simulink model "gm_hdlcoder_led_blinking_4bit_interface"  (R2021b)
settings: Solver=FixedStepDiscrete  StartTime=0.0  StopTime=inf  RelTol=1e-3  EnableMultiTasking=on
InitFcn:
  | Ts = 1e-3;
undefined symbols (not defined in the file or in its folder): AXI4, Lite
libraries: axiinterfacelib x3, simulink x2
settings Model: Creator=The MathWorks, Inc.  LastModifiedBy=Jeedella
settings SolverCC: ConcurrentTasks=on  AlgebraicLoopSolver=TrustRegion  PositivePriorityOrder=on
settings DataIOCC: LimitDataPoints=on  SaveFormat=Array  SaveOutput=off  SignalLogging=off  SaveTime=off  ReturnWorkspaceOutputs=off
settings OptimizationCC: BlockReduction=off  ConditionallyExecuteInputs=off  EnhancedBackFolding=on  PassReuseOutputArgsAs=Individual arguments  ExpressionDepthLimit=2147483647  ZeroExternalMemoryAtStartup=off  ZeroInternalMemoryAtStartup=off  MaxStackSize=64  OptimizeBlockOrder=speed  DifferentSizesBufferReuse=on  OptimizationCustomize=off  EfficientTunableParamExpr=on
settings DebuggingCC: AlgebraicLoopMsg=error  UnderspecifiedInitializationDetection=Classic  MergeDetectMultiDrivingBlocksExec=none  SolverPrmCheckMsg=warning  SingleTaskRateTransMsg=error  ParameterPrecisionLossMsg=none  ParameterTunabilityLossMsg=error  StateNameClashWarn=warning  SFUnexpectedBacktrackingDiag=warning  SFNoUnconditionalDefaultTransitionDiag=warning  SFExecutionAtInitializationDiag=none  SFMachineParentedDataDiag=warning  ArithmeticOperatorsInVariantConditions=warning
settings HardwareCC: ProdBitPerPointer=32  ProdBitPerSizeT=32  ProdBitPerPtrDiffT=32  ProdLargestAtomicInteger=Long  ProdLargestAtomicFloat=Double  ProdWordSize=32  ProdLongLongMode=on  ProdHWDeviceType=ARM Compatible->ARM Cortex  TargetEndianess=LittleEndian
settings ModelReferenceCC: ModelReferenceNumInstancesAllowed=Single  PropagateSignalLabelsOutOfModel=off
settings SFSimCC: SimUseLocalCustomCode=off  MATLABDynamicMemAlloc=off  CustomCodeUndefinedFunction=UseInterfaceOnly
settings RTWCC: Description=Embedded Coder  SystemTargetFile=ert.tlc  HardwareBoard=Xilinx Zynq-7000 based board  TLCOptions="-aInlineSetEventsForThisBaseRateFcn=TLC_FALSE -aSuppressMultiTaskScheduler=TLC_FALSE  -aRateBasedStepFcn=0"  TemplateMakefile=ert_default_tmf  RTWUseLocalCustomCode=off  Toolchain=Linaro AArch32 Linux v6.3.1
settings CodeAppCC: ForceParamTrailComments=on  IgnoreCustomStorageClasses=off  OperatorAnnotations=on  SimulinkDataObjDesc=on  SFDataObjDesc=on  InsertBlockDesc=on
settings ConfigComp: CovMetricSettings=dw  CovSaveCumulativeToWorkspaceVar=on  CovSaveSingleToWorkspaceVar=on  CovExternalEMLEnable=off  CovSFcnEnable=off

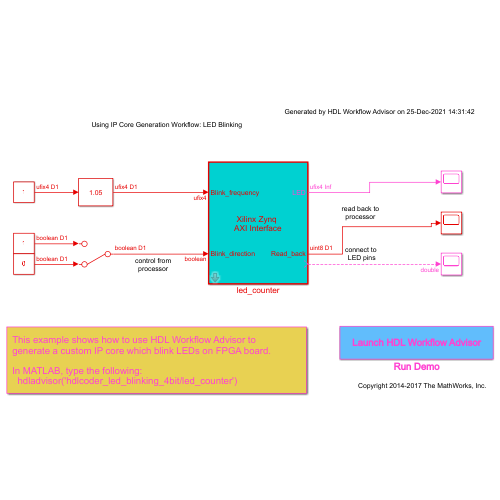
[thumbnail: Simulink's stored preview of the top-level diagram]
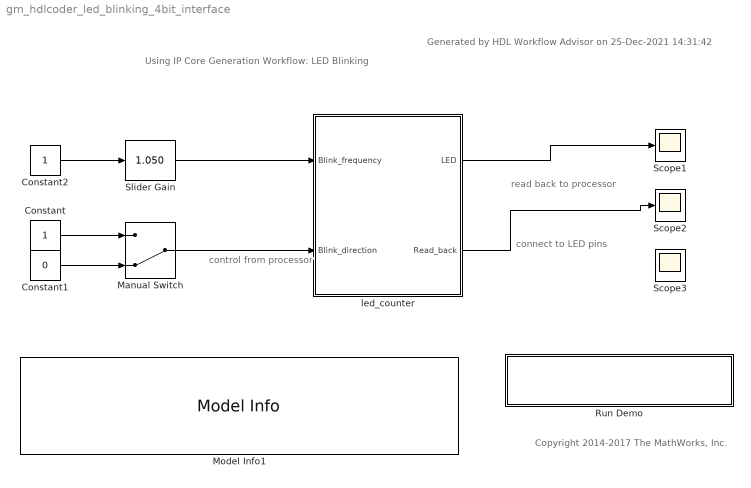
== system gm_hdlcoder_led_blinking_4bit_interface ==
  note: connect to
      | LED pins
  note: read back to
      | processor
  note: control from
      | processor
  note: Using IP Core Generation Workflow: LED Blinking
  note: Copyright 2014-2017 The MathWorks, Inc.
  note: Generated by HDL Workflow Advisor on 25-Dec-2021 14:31:42
  Constant : Constant  OutDataTypeStr=boolean  SampleTime=Ts
  Constant1 : Constant  Value=0  OutDataTypeStr=boolean  SampleTime=Ts
  Constant2 : Constant  OutDataTypeStr=fixdt(0, 4, 0)  SampleTime=Ts
  Manual Switch : ManualSwitch  CurrentSetting=0
  Model Info1 : simulink/Model-Wide Utilities/Model Info  Frame=on  DisplayStringWithTags=|  HorizontalTextAlignment=Left  LeftAlignmentValue=0.02
      | This example shows how to use HDL Workflow Advisor to    
      | generate a custom IP core which blink LEDs on FPGA board.
      |                                                          
      | In MATLAB, type the following:                           
      |   hdladvisor('hdlcoder_led_blinking_4bit/led_counter')
  Run Demo : Subsystem
      settings: OpenFcn=hdladvisor([bdroot, '/led_counter'])
      mask Display: disp('Launch HDL Workflow Advisor')
  Scope1 : Scope
  Scope2 : Scope
  Scope3 : Scope
  Slider Gain : simulink/Math Operations/Slider Gain  gain=1.050  low=0  high=15
  led_counter : Subsystem  TreatAsAtomicUnit=on  mask(AXI4-Lite/AXI4 Interface){}
      mask help:
      | This is an automatically generated subsystem block.
      | This contains the AXI interface blocks that communicate with the led_count_ip IPCore generated from hdlcoder_led_blinking_4bit/led_counter subsystem.
      mask Display: disp(sprintf('Xilinx Zynq \nAXI Interface'));
  wires:
  ? -> Scope3/1
  led_counter/1(LED) -> Scope1/1
  led_counter/2(Read_back) -> Scope2/1
  Slider Gain/1 -> led_counter/1(Blink_frequency)
  Constant2/1 -> Slider Gain/1
  Manual Switch/1 -> led_counter/2(Blink_direction)
  Constant1/1 -> Manual Switch/2
  Constant/1 -> Manual Switch/1

== system gm_hdlcoder_led_blinking_4bit_interface/Run Demo ==

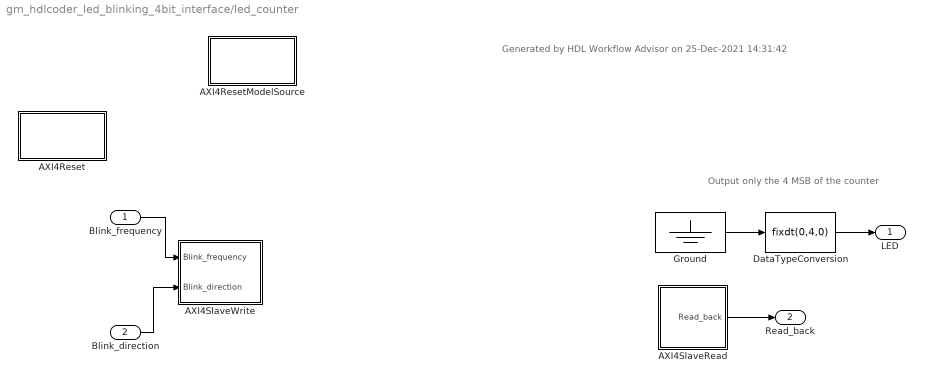
== system gm_hdlcoder_led_blinking_4bit_interface/led_counter ==
  note: Output only the 4 MSB of the counter
  note: Generated by HDL Workflow Advisor on 25-Dec-2021 14:31:42
  Blink_frequency : Inport  OutDataTypeStr=fixdt(0, 4, 0)
  Blink_direction : Inport  Port=2  OutDataTypeStr=boolean
  AXI4Reset : Subsystem  mask(System Start){ShowInLibBrowser=0}
      mask prompts: ShowInLibBrowser "Simulink:masks:CustCodeMaskParam1_MP"
      settings: CopyFcn=cccopyfcn(gcb)  OpenFcn=ccopenfcn('System Start Function')
      mask Help: eval('feval(''rtwprivate'',''rtwhelpview'',''rtw_sys_start_block'')');
      mask Display: disp('System\nStart');
  AXI4ResetModelSource : Subsystem  mask(Model Source){ShowInLibBrowser=0}
      mask prompts: ShowInLibBrowser "Simulink:masks:CustCodeMaskParam1_MP"
      settings: CopyFcn=cccopyfcn(gcb)  OpenFcn=ccopenfcn('Model Source')
      mask Help: eval('feval(''rtwprivate'',''rtwhelpview'',''rtw_model_source_block'')');
      mask Display: disp('Model\nSource');
  AXI4SlaveRead : Subsystem  Priority=10
  AXI4SlaveWrite : Subsystem  Priority=1
  DataTypeConversion : DataTypeConversion  OutDataTypeStr=fixdt(0,4,0)  ConvertRealWorld=Stored Integer (SI)
  Ground : Ground
  LED : Outport  VectorParamsAs1DForOutWhenUnconnected=off
  Read_back : Outport  Port=2  VectorParamsAs1DForOutWhenUnconnected=off
  wires:
  Blink_frequency/1 -> AXI4SlaveWrite/1(Blink_frequency)
  Blink_direction/1 -> AXI4SlaveWrite/2(Blink_direction)
  AXI4SlaveRead/1(Read_back) -> Read_back/1
  DataTypeConversion/1 -> LED/1
  Ground/1 -> DataTypeConversion/1

== system gm_hdlcoder_led_blinking_4bit_interface/led_counter/AXI4Reset ==

== system gm_hdlcoder_led_blinking_4bit_interface/led_counter/AXI4ResetModelSource ==

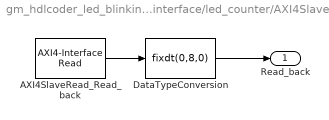
== system gm_hdlcoder_led_blinking_4bit_interface/led_counter/AXI4SlaveRead ==
  AXI4SlaveRead_Read_back : axiinterfacelib/AXI4-Interface Read  Priority=3  AXIInterfaceType=AXI4-Lite  DeviceName=/dev/mwipcore  RegisterOffset=hex2dec('108')  DataLength=1  DataType=uint32  SampleTime=-1  blockPlatform=ZYNQ  SimulateUsing=Interpreted Execution
      settings: SourceProductBaseCode=ECZYNQ7000
  DataTypeConversion : DataTypeConversion  OutDataTypeStr=fixdt(0,8,0)  ConvertRealWorld=Stored Integer (SI)
  Read_back : Outport  VectorParamsAs1DForOutWhenUnconnected=off
  wires:
  DataTypeConversion/1 -> Read_back/1
  AXI4SlaveRead_Read_back/1 -> DataTypeConversion/1

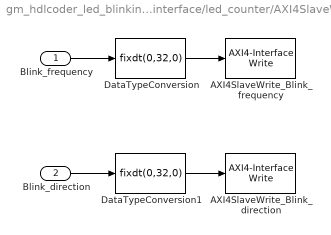
== system gm_hdlcoder_led_blinking_4bit_interface/led_counter/AXI4SlaveWrite ==
  Blink_frequency : Inport  OutDataTypeStr=fixdt(0, 4, 0)
  Blink_direction : Inport  Port=2  OutDataTypeStr=boolean
  AXI4SlaveWrite_Blink_direction : axiinterfacelib/AXI4-Interface Write  Priority=3  AXIInterfaceType=AXI4-Lite  DeviceName=/dev/mwipcore  RegisterOffset=hex2dec('104')  blockPlatform=ZYNQ  SimulateUsing=Interpreted execution
      settings: SourceProductBaseCode=ECZYNQ7000
  AXI4SlaveWrite_Blink_frequency : axiinterfacelib/AXI4-Interface Write  Priority=2  AXIInterfaceType=AXI4-Lite  DeviceName=/dev/mwipcore  RegisterOffset=hex2dec('100')  blockPlatform=ZYNQ  SimulateUsing=Interpreted execution
      settings: SourceProductBaseCode=ECZYNQ7000
  DataTypeConversion : DataTypeConversion  OutDataTypeStr=fixdt(0,32,0)  ConvertRealWorld=Stored Integer (SI)
  DataTypeConversion1 : DataTypeConversion  OutDataTypeStr=fixdt(0,32,0)  ConvertRealWorld=Stored Integer (SI)
  wires:
  Blink_direction/1 -> DataTypeConversion1/1
  DataTypeConversion1/1 -> AXI4SlaveWrite_Blink_direction/1
  Blink_frequency/1 -> DataTypeConversion/1
  DataTypeConversion/1 -> AXI4SlaveWrite_Blink_frequency/1
